simulink model "LQ_Luenberger_no_obs"  (R2023b)
settings: Solver=VariableStepAuto  StartTime=0.0  StopTime=10.0  RelTol=1e-3
values from neighbouring files (symbols this model uses):
  Ken_eta = K(:, 4)    [LQ_KF.m]    (also in LQ_KF_version1.m; LQ_KF_version2.m = Ken(:, n+1:end); LQ_Luenberger.m; LQ_prova.m = Ken(:, n+1:end))
  Ken_x = K(:, 1:3)    [LQ_KF.m]    (also in LQ_KF_version1.m; LQ_KF_version2.m = Ken(:, 1:n); LQ_Luenberger.m; LQ_prova.m = Ken(:, 1:n))
undefined symbols (not defined in the file or in its folder): Lc, Rtot, x1_eq0, x2_eq0, x3_eq0
libraries: simulink x1
settings Model: Creator=Pronto all'uso  LastModifiedBy=Pronto all'uso

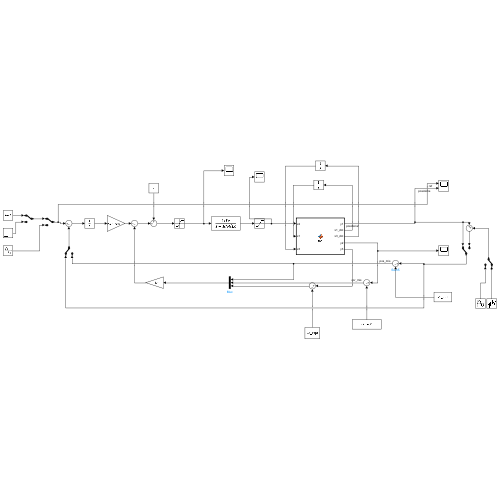
[thumbnail: Simulink's stored preview of the top-level diagram]
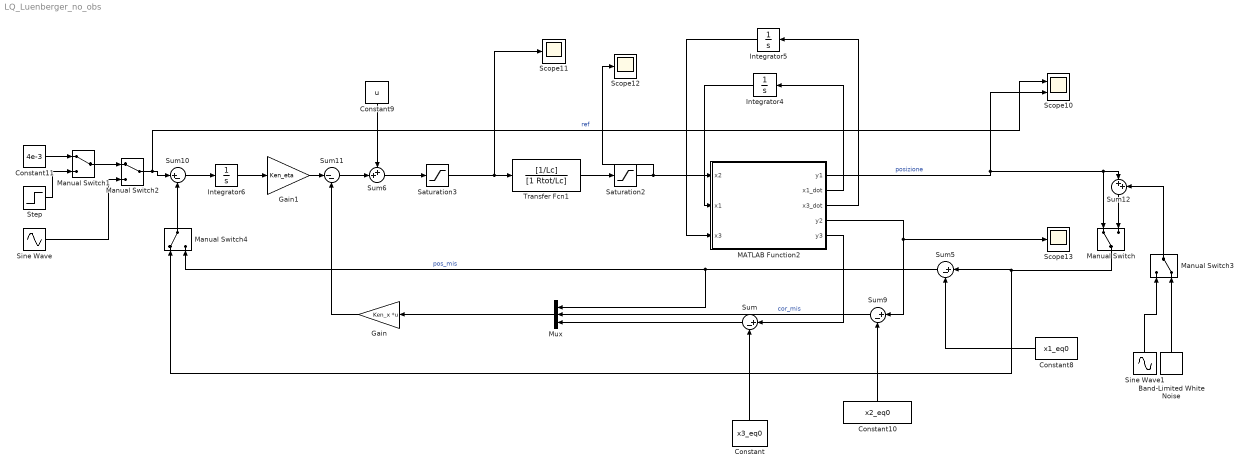
== system LQ_Luenberger_no_obs ==
  Band-Limited White Noise : simulink/Sources/Band-Limited White Noise  Cov=[8.9934e-11*0.002]  Ts=0.002  seed=[23341]
  Constant : Constant  Value=x3_eq0
  Constant10 : Constant  Value=x2_eq0
  Constant11 : Constant  Value=4e-3
  Constant8 : Constant  Value=x1_eq0
  Constant9 : Constant  Value=u
  Gain : Gain  Gain=Ken_x  Multiplication=Matrix(K*u)
  Gain1 : Gain  Gain=Ken_eta
  Integrator4 : Integrator
  Integrator5 : Integrator
  Integrator6 : Integrator
  MATLAB Function2 : MATLAB Function  TreatAsAtomicUnit=on
  Manual Switch{,1..2,4} (4 alike) : ManualSwitch
  Manual Switch3 : ManualSwitch  CurrentSetting=0
  Mux : Mux  Inputs=3
  Saturation2 : Saturate  UpperLimit=3  LowerLimit=0
  Saturation3 : Saturate  UpperLimit=24  LowerLimit=-24
  Scope10 : Scope  NumInputPorts=2
  Scope11 : Scope
  Scope12 : Scope
  Scope13 : Scope
  Sine Wave : Sin  Amplitude=0.001  Bias=0.005  SampleTime=0
  Sine Wave1 : Sin  Amplitude=0.00001  Frequency=200  SampleTime=0.002
  Step : Step  Time=3  After=0.001  SampleTime=0
  Sum{,5,9..10} (4 alike) : Sum  Inputs=|+-
  Sum11 : Sum  Inputs=|--
  Sum12 : Sum  Inputs=|++
  Sum6 : Sum  Inputs=++|
  Transfer Fcn1 : TransferFcn  Numerator=[1/Lc]  Denominator=[1 Rtot/Lc]
  wires:
  Integrator5/1 -> MATLAB Function2/3(x3)
  Manual Switch4/1 -> Sum10/2
  MATLAB Function2/3(x3_dot) -> Integrator5/1
  Transfer Fcn1/1 -> Saturation2/1
  Constant10/1 -> Sum9/2
  Step/1 -> Manual Switch1/2
  Sum11/1 -> Sum6/2
  Constant11/1 -> Manual Switch1/1
  Integrator6/1 -> Gain1/1
  Manual Switch3/1 -> Sum12/2
  Saturation2/1 -> MATLAB Function2/1(x2), Scope12/1
  Manual Switch1/1 -> Manual Switch2/1
  Sum6/1 -> Saturation3/1
  MATLAB Function2/1(y1) -> Manual Switch/1, Sum12/1, Scope10/2  "posizione"
  Sum12/1 -> Manual Switch/2
  Band-Limited White Noise/1 -> Manual Switch3/2
  Manual Switch/1 -> Manual Switch4/1, Sum5/1
  Integrator4/1 -> MATLAB Function2/2(x1)
  Constant8/1 -> Sum5/2
  Sine Wave/1 -> Manual Switch2/2
  MATLAB Function2/4(y2) -> Sum9/1, Scope13/1
  Manual Switch2/1 -> Scope10/1, Sum10/1  "ref"
  Constant9/1 -> Sum6/1
  Gain1/1 -> Sum11/1
  Sine Wave1/1 -> Manual Switch3/1
  Sum9/1 -> Mux/2  "cor_mis"
  Gain/1 -> Sum11/2
  MATLAB Function2/2(x1_dot) -> Integrator4/1
  Sum5/1 -> Mux/1, Manual Switch4/2  "pos_mis"
  Sum10/1 -> Integrator6/1
  Saturation3/1 -> Transfer Fcn1/1, Scope11/1
  Mux/1 -> Gain/1
  MATLAB Function2/5(y3) -> Sum/1
  Constant/1 -> Sum/2
  Sum/1 -> Mux/3

== matlab function LQ_Luenberger_no_obs/MATLAB Function2 ==
  data: y1 output; x2 input; x1_dot output; x1 input; x3 input; x3_dot output; y2 output; y3 output
function [y1,x1_dot, x3_dot, y2, y3] = fcn(x2, x1, x3)
    m = 0.0657;
    g = 9.81;
    k_mag = 2.4405e-05;
    Rtot = 9.7585;
    Lc = 0.3708;
    y0 = 0.012;
    
    x1_dot = x3;
    x3_dot = (k_mag/m)*(x2/(y0-x1))^2 - g;

    if x1 <= 0 && x3_dot < 0
        x1 = 0;
        x3 = 0;
        x3_dot = 0;
    end
y1 = x1;
y2 = x2;
y3 = x3;
